simulink model "Ornek3_14"  (R2021b)
settings: Solver=VariableStepAuto  StartTime=0.0  StopTime=9  RelTol=1e-3
libraries: dspquant2 x2, dspsigops x1
settings Model: Creator=MONSTER  LastModifiedBy=MONSTER

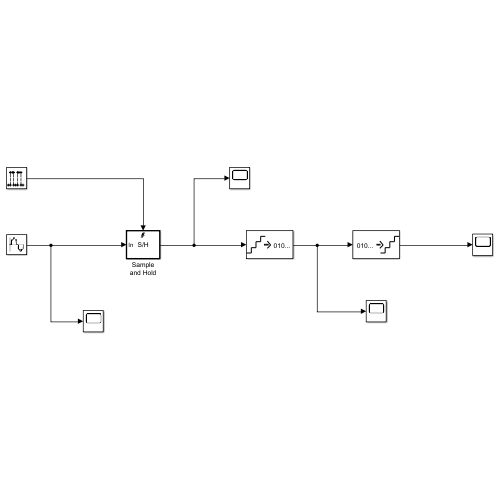
[thumbnail: Simulink's stored preview of the top-level diagram]
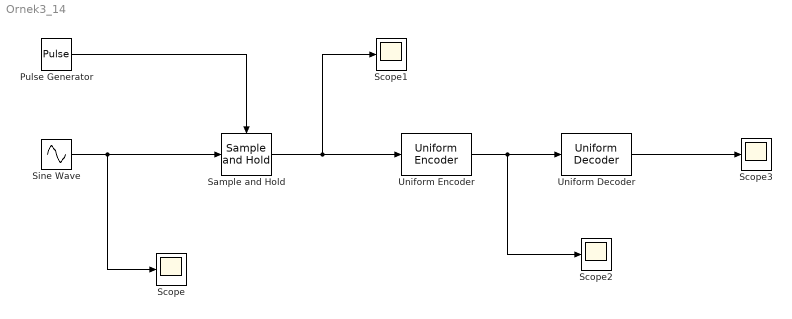
== system Ornek3_14 ==
  Pulse Generator : DiscretePulseGenerator  Period=9  PulseWidth=4  SampleTime=0.001
  Sample and Hold : dspsigops/Sample and Hold  trig=Rising edge  initCond=0  latchinput=off
  Scope{,1..3} (4 alike) : Scope
  Sine Wave : Sin  SampleTime=0.001
  Uniform Decoder : dspquant2/Uniform Decoder  peak=1  bits=8  overflowMode=Saturate  otype=Double
      settings: SourceProductBaseCode=DS
  Uniform Encoder : dspquant2/Uniform Encoder  peak=1  bits=8  otype=Unsigned integer
  wires:
  Pulse Generator/1 -> Sample and Hold/Trigger
  Sine Wave/1 -> Scope/1, Sample and Hold/1
  Sample and Hold/1 -> Scope1/1, Uniform Encoder/1
  Uniform Encoder/1 -> Scope2/1, Uniform Decoder/1
  Uniform Decoder/1 -> Scope3/1
